simulink model "State_Space_Nominal"  (R2021a)
settings: Solver=ode45  StartTime=0.0  StopTime=20  RelTol=1e-3
undefined symbols (not defined in the file): degs2rpm, drv, est_par, gbox, mot, nominal, rads2rpm, rpm2rads, sens
settings Model: Creator=Utente  LastModifiedBy=gioel
settings SolverCC: AlgebraicLoopSolver=TrustRegion
settings DataIOCC: ReturnWorkspaceOutputs=off
settings DebuggingCC: SFMachineParentedDataDiag=warning

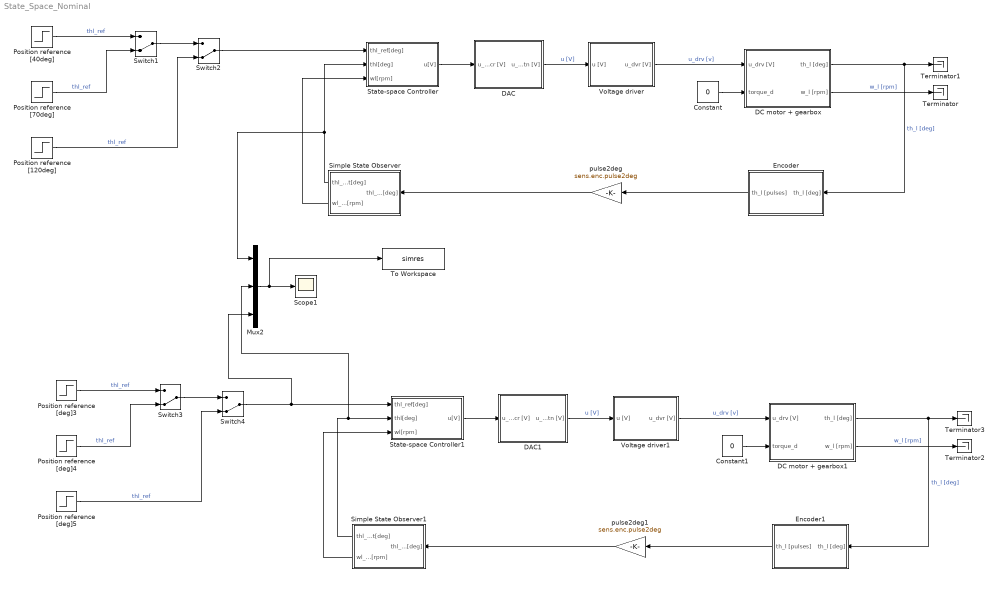
== system State_Space_Nominal ==
  Constant : Constant  Value=0
  Constant1 : Constant  Value=0
  DAC : Subsystem
  DAC1 : Subsystem
  DC motor + gearbox : Subsystem
  DC motor + gearbox1 : Subsystem
  Encoder : Subsystem
  Encoder1 : Subsystem
  Mux2 : Mux  Inputs=3
  Position reference [120deg] : Step  Time=0  After=120  SampleTime=0
  Position reference [40deg] : Step  Time=0  After=40  SampleTime=0
  Position reference [70deg] : Step  Time=0  After=70  SampleTime=0
  Position reference [deg]3 : Step  Time=0  After=40  SampleTime=0
  Position reference [deg]4 : Step  Time=0  After=70  SampleTime=0
  Position reference [deg]5 : Step  Time=0  After=120  SampleTime=0
  Scope1 : Scope
  Simple State Observer : Subsystem
  Simple State Observer1 : Subsystem
  State-space Controller : Subsystem
  State-space Controller1 : Subsystem
  Switch{1..4} (4 alike) : ManualSwitch  CurrentSetting=0
  Terminator{,1..3} (4 alike) : Terminator
  To Workspace : ToWorkspace  VariableName=simres  SaveFormat=Structure With Time  SampleTime=-1
  Voltage driver : Subsystem
  Voltage driver1 : Subsystem
  pulse2deg : Gain  Gain=sens.enc.pulse2deg
  pulse2deg1 : Gain  Gain=sens.enc.pulse2deg
  wires:
  DAC/1(u_cntn [V]) -> Voltage driver/1(u [V])  "u [V]"
  Voltage driver/1(u_dvr [V]) -> DC motor + gearbox/1(u_drv [V])  "u_drv [v]"
  Constant/1 -> DC motor + gearbox/2(torque_d)
  pulse2deg/1 -> Simple State Observer/1(thl_meas[deg])
  Encoder/1(th_l [pulses]) -> pulse2deg/1
  DC motor + gearbox/1(th_l [deg]) -> Terminator1/1, Encoder/1(th_l [deg])  "th_l [deg]"
  DC motor + gearbox/2(w_l [rpm]) -> Terminator/1  "w_l [rpm]"
  Switch2/1 -> State-space Controller/1(thl_ref[deg])
  Position reference [40deg]/1 -> Switch1/1  "thl_ref"
  Position reference [70deg]/1 -> Switch1/2  "thl_ref"
  Switch1/1 -> Switch2/1
  Position reference [120deg]/1 -> Switch2/2  "thl_ref"
  pulse2deg1/1 -> Simple State Observer1/1(thl_meas[deg])
  Switch3/1 -> Switch4/1
  DAC1/1(u_cntn [V]) -> Voltage driver1/1(u [V])  "u [V]"
  Position reference [deg]3/1 -> Switch3/1  "thl_ref"
  Simple State Observer1/2(wl_est[rpm]) -> State-space Controller1/3(wl[rpm])
  Voltage driver1/1(u_dvr [V]) -> DC motor + gearbox1/1(u_drv [V])  "u_drv [v]"
  Position reference [deg]5/1 -> Switch4/2  "thl_ref"
  Switch4/1 -> Mux2/3, State-space Controller1/1(thl_ref[deg])
  Encoder1/1(th_l [pulses]) -> pulse2deg1/1
  Constant1/1 -> DC motor + gearbox1/2(torque_d)
  DC motor + gearbox1/2(w_l [rpm]) -> Terminator2/1  "w_l [rpm]"
  State-space Controller1/1(u[V]) -> DAC1/1(u_dscr [V])
  DC motor + gearbox1/1(th_l [deg]) -> Terminator3/1, Encoder1/1(th_l [deg])  "th_l [deg]"
  Position reference [deg]4/1 -> Switch3/2  "thl_ref"
  Simple State Observer/1(thl_est[deg]) -> State-space Controller/2(thl[deg]), Mux2/1
  Simple State Observer/2(wl_est[rpm]) -> State-space Controller/3(wl[rpm])
  State-space Controller/1(u[V]) -> DAC/1(u_dscr [V])
  Simple State Observer1/1(thl_est[deg]) -> Mux2/2, State-space Controller1/2(thl[deg])
  Mux2/1 -> To Workspace/1, Scope1/1

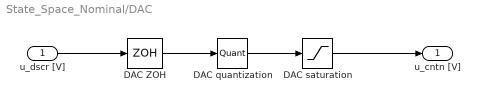
== system State_Space_Nominal/DAC ==
  u_dscr [V] : Inport
  DAC ZOH : ZeroOrderHold  SampleTime=sens.enc.T_s
  DAC quantization : Quantizer  QuantizationInterval=daq.dac.q
  DAC saturation : Saturate  UpperLimit=10  LowerLimit=-10
  u_cntn [V] : Outport
  wires:
  DAC quantization/1 -> DAC saturation/1
  DAC ZOH/1 -> DAC quantization/1
  DAC saturation/1 -> u_cntn [V]/1
  u_dscr [V]/1 -> DAC ZOH/1

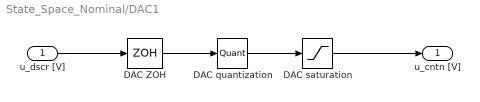
== system State_Space_Nominal/DAC1 ==
  u_dscr [V] : Inport
  DAC ZOH : ZeroOrderHold  SampleTime=sens.enc.T_s
  DAC quantization : Quantizer  QuantizationInterval=daq.dac.q
  DAC saturation : Saturate  UpperLimit=10  LowerLimit=-10
  u_cntn [V] : Outport
  wires:
  DAC quantization/1 -> DAC saturation/1
  DAC ZOH/1 -> DAC quantization/1
  DAC saturation/1 -> u_cntn [V]/1
  u_dscr [V]/1 -> DAC ZOH/1

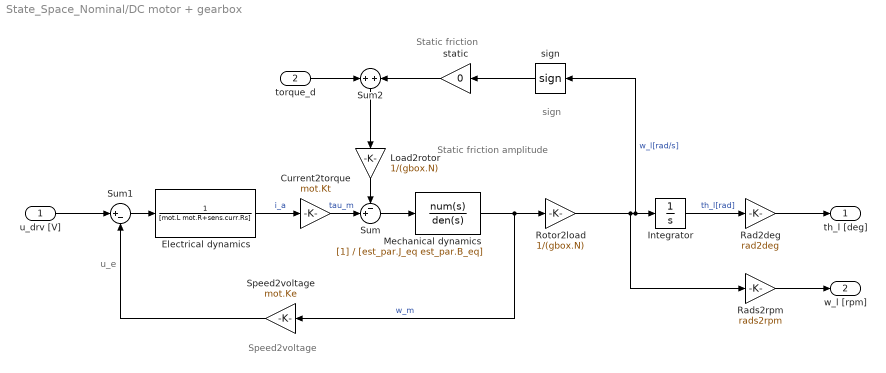
== system State_Space_Nominal/DC motor + gearbox ==
  note: u_e
  note: Speed2voltage
  note: Static friction
  note: sign
  note: Static friction
      |  amplitude
  u_drv [V] : Inport
  torque_d : Inport  Port=2
  Current2torque : Gain  Gain=mot.Kt
  Electrical dynamics : TransferFcn  Denominator=[mot.L mot.R+sens.curr.Rs]
  Integrator : Integrator
  Load2rotor : Gain  Gain=1/(gbox.N)
  Mechanical dynamics : TransferFcn  Denominator=[est_par.J_eq est_par.B_eq]
  Rad2deg : Gain  Gain=rad2deg
  Rads2rpm : Gain  Gain=rads2rpm
  Rotor2load : Gain  Gain=1/(gbox.N)
  Speed2voltage : Gain  Gain=mot.Ke
  Sum : Sum  Inputs=-+|
  Sum1 : Sum  Inputs=|+-
  Sum2 : Sum  Inputs=+|+
  sign : Signum  ZeroCross=off
  static : Gain  Gain=0
  th_l [deg] : Outport
  w_l [rpm] : Outport  Port=2
  wires:
  u_drv [V]/1 -> Sum1/1
  Rads2rpm/1 -> w_l [rpm]/1
  Electrical dynamics/1 -> Current2torque/1  "i_a"
  Current2torque/1 -> Sum/2  "tau_m"
  Rad2deg/1 -> th_l [deg]/1
  sign/1 -> static/1
  Sum1/1 -> Electrical dynamics/1
  Integrator/1 -> Rad2deg/1  "th_l[rad]"
  Sum/1 -> Mechanical dynamics/1
  Load2rotor/1 -> Sum/1
  Speed2voltage/1 -> Sum1/2
  Rotor2load/1 -> sign/1, Integrator/1, Rads2rpm/1  "w_l[rad/s]"
  Mechanical dynamics/1 -> Speed2voltage/1, Rotor2load/1  "w_m"
  Sum2/1 -> Load2rotor/1
  torque_d/1 -> Sum2/1
  static/1 -> Sum2/2

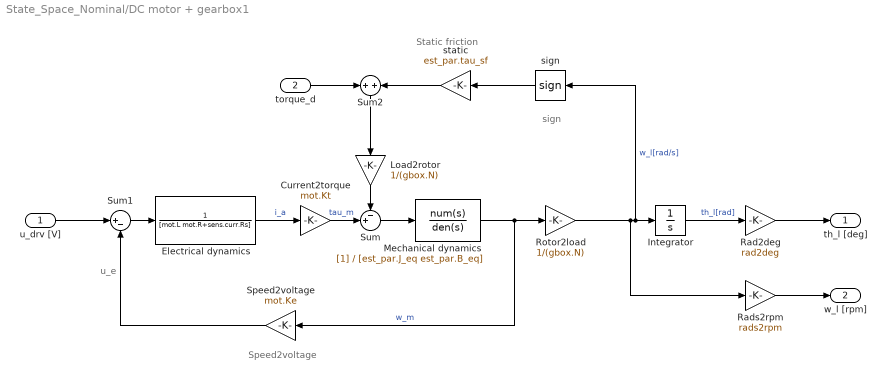
== system State_Space_Nominal/DC motor + gearbox1 ==
  note: u_e
  note: Speed2voltage
  note: Static friction
  note: sign
  u_drv [V] : Inport
  torque_d : Inport  Port=2
  Current2torque : Gain  Gain=mot.Kt
  Electrical dynamics : TransferFcn  Denominator=[mot.L mot.R+sens.curr.Rs]
  Integrator : Integrator
  Load2rotor : Gain  Gain=1/(gbox.N)
  Mechanical dynamics : TransferFcn  Denominator=[est_par.J_eq est_par.B_eq]
  Rad2deg : Gain  Gain=rad2deg
  Rads2rpm : Gain  Gain=rads2rpm
  Rotor2load : Gain  Gain=1/(gbox.N)
  Speed2voltage : Gain  Gain=mot.Ke
  Sum : Sum  Inputs=-+|
  Sum1 : Sum  Inputs=|+-
  Sum2 : Sum  Inputs=+|+
  sign : Signum  ZeroCross=off
  static : Gain  Gain=est_par.tau_sf
  th_l [deg] : Outport
  w_l [rpm] : Outport  Port=2
  wires:
  u_drv [V]/1 -> Sum1/1
  Rads2rpm/1 -> w_l [rpm]/1
  Electrical dynamics/1 -> Current2torque/1  "i_a"
  Current2torque/1 -> Sum/2  "tau_m"
  Rad2deg/1 -> th_l [deg]/1
  sign/1 -> static/1
  Sum1/1 -> Electrical dynamics/1
  Integrator/1 -> Rad2deg/1  "th_l[rad]"
  Sum/1 -> Mechanical dynamics/1
  Load2rotor/1 -> Sum/1
  Speed2voltage/1 -> Sum1/2
  Rotor2load/1 -> sign/1, Integrator/1, Rads2rpm/1  "w_l[rad/s]"
  Mechanical dynamics/1 -> Speed2voltage/1, Rotor2load/1  "w_m"
  Sum2/1 -> Load2rotor/1
  torque_d/1 -> Sum2/1
  static/1 -> Sum2/2

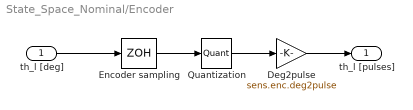
== system State_Space_Nominal/Encoder ==
  th_l [deg] : Inport
  Deg2pulse : Gain  Gain=sens.enc.deg2pulse
  Encoder sampling : ZeroOrderHold  SampleTime=0.001
  Quantization : Quantizer  QuantizationInterval=sens.enc.q
  th_l [pulses] : Outport
  wires:
  Encoder sampling/1 -> Quantization/1
  Quantization/1 -> Deg2pulse/1
  th_l [deg]/1 -> Encoder sampling/1
  Deg2pulse/1 -> th_l [pulses]/1

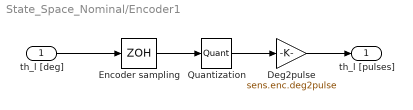
== system State_Space_Nominal/Encoder1 ==
  th_l [deg] : Inport
  Deg2pulse : Gain  Gain=sens.enc.deg2pulse
  Encoder sampling : ZeroOrderHold  SampleTime=0.001
  Quantization : Quantizer  QuantizationInterval=sens.enc.q
  th_l [pulses] : Outport
  wires:
  Encoder sampling/1 -> Quantization/1
  Quantization/1 -> Deg2pulse/1
  th_l [deg]/1 -> Encoder sampling/1
  Deg2pulse/1 -> th_l [pulses]/1

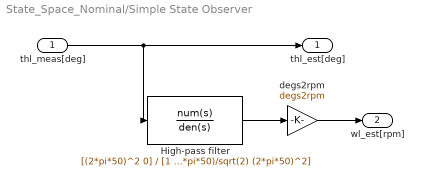
== system State_Space_Nominal/Simple State Observer ==
  thl_meas[deg] : Inport
  High-pass filter : TransferFcn  Numerator=[(2*pi*50)^2 0]  Denominator=[1 (2*2*pi*50)/sqrt(2) (2*pi*50)^2]
  degs2rpm : Gain  Gain=degs2rpm
  thl_est[deg] : Outport
  wl_est[rpm] : Outport  Port=2
  wires:
  High-pass filter/1 -> degs2rpm/1
  degs2rpm/1 -> wl_est[rpm]/1
  thl_meas[deg]/1 -> thl_est[deg]/1, High-pass filter/1

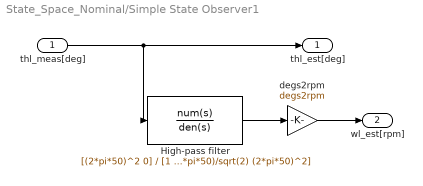
== system State_Space_Nominal/Simple State Observer1 ==
  thl_meas[deg] : Inport
  High-pass filter : TransferFcn  Numerator=[(2*pi*50)^2 0]  Denominator=[1 (2*2*pi*50)/sqrt(2) (2*pi*50)^2]
  degs2rpm : Gain  Gain=degs2rpm
  thl_est[deg] : Outport
  wl_est[rpm] : Outport  Port=2
  wires:
  High-pass filter/1 -> degs2rpm/1
  degs2rpm/1 -> wl_est[rpm]/1
  thl_meas[deg]/1 -> thl_est[deg]/1, High-pass filter/1

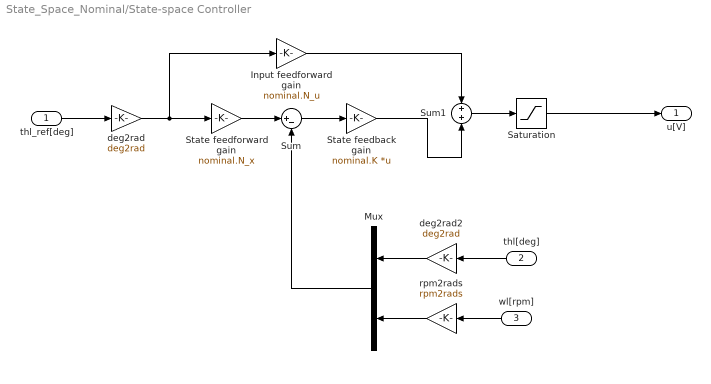
== system State_Space_Nominal/State-space Controller ==
  thl_ref[deg] : Inport
  thl[deg] : Inport  Port=2
  wl[rpm] : Inport  Port=3
  Input feedforward gain : Gain  Gain=nominal.N_u
  Mux : Mux  Inputs=2
  Saturation : Saturate  UpperLimit=10  LowerLimit=-10
  State feedback gain : Gain  Gain=nominal.K  Multiplication=Matrix(K*u)
  State feedforward gain : Gain  Gain=nominal.N_x
  Sum : Sum  Inputs=|+-
  Sum1 : Sum
  deg2rad : Gain  Gain=deg2rad
  deg2rad2 : Gain  Gain=deg2rad
  rpm2rads : Gain  Gain=rpm2rads
  u[V] : Outport
  wires:
  rpm2rads/1 -> Mux/2
  thl_ref[deg]/1 -> deg2rad/1
  wl[rpm]/1 -> rpm2rads/1
  deg2rad/1 -> Input feedforward gain/1, State feedforward gain/1
  thl[deg]/1 -> deg2rad2/1
  Saturation/1 -> u[V]/1
  State feedforward gain/1 -> Sum/1
  Sum/1 -> State feedback gain/1
  Mux/1 -> Sum/2
  deg2rad2/1 -> Mux/1
  Sum1/1 -> Saturation/1
  Input feedforward gain/1 -> Sum1/1
  State feedback gain/1 -> Sum1/2

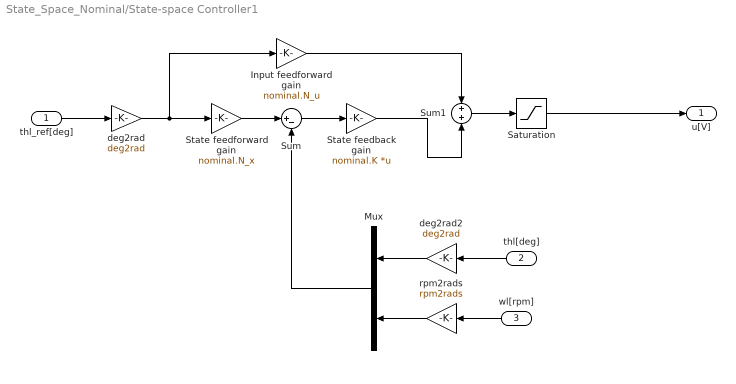
== system State_Space_Nominal/State-space Controller1 ==
  thl_ref[deg] : Inport
  thl[deg] : Inport  Port=2
  wl[rpm] : Inport  Port=3
  Input feedforward gain : Gain  Gain=nominal.N_u
  Mux : Mux  Inputs=2
  Saturation : Saturate  UpperLimit=10  LowerLimit=-10
  State feedback gain : Gain  Gain=nominal.K  Multiplication=Matrix(K*u)
  State feedforward gain : Gain  Gain=nominal.N_x
  Sum : Sum  Inputs=|+-
  Sum1 : Sum
  deg2rad : Gain  Gain=deg2rad
  deg2rad2 : Gain  Gain=deg2rad
  rpm2rads : Gain  Gain=rpm2rads
  u[V] : Outport
  wires:
  thl[deg]/1 -> deg2rad2/1
  Sum/1 -> State feedback gain/1
  rpm2rads/1 -> Mux/2
  State feedback gain/1 -> Sum1/2
  Sum1/1 -> Saturation/1
  Input feedforward gain/1 -> Sum1/1
  Mux/1 -> Sum/2
  deg2rad/1 -> Input feedforward gain/1, State feedforward gain/1
  deg2rad2/1 -> Mux/1
  wl[rpm]/1 -> rpm2rads/1
  State feedforward gain/1 -> Sum/1
  thl_ref[deg]/1 -> deg2rad/1
  Saturation/1 -> u[V]/1

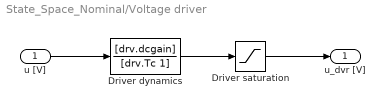
== system State_Space_Nominal/Voltage driver ==
  u [V] : Inport
  Driver dynamics : TransferFcn  Numerator=[drv.dcgain]  Denominator=[drv.Tc 1]
  Driver saturation : Saturate  UpperLimit=12  LowerLimit=-12
  u_dvr [V] : Outport
  wires:
  Driver saturation/1 -> u_dvr [V]/1
  Driver dynamics/1 -> Driver saturation/1
  u [V]/1 -> Driver dynamics/1

== system State_Space_Nominal/Voltage driver1 ==
  u [V] : Inport
  Driver dynamics : TransferFcn  Numerator=[drv.dcgain]  Denominator=[drv.Tc 1]
  Driver saturation : Saturate  UpperLimit=12  LowerLimit=-12
  u_dvr [V] : Outport
  wires:
  Driver saturation/1 -> u_dvr [V]/1
  Driver dynamics/1 -> Driver saturation/1
  u [V]/1 -> Driver dynamics/1
